simulink model "Test_driver"  (Simulink 7.6)
settings: Solver=ode45  StartTime=0.0  StopTime=10.0  RelTol=1e-3
undefined symbols (not defined in the file): Battery_Initial_Percentage, Battery_Nominal_Voltage, Battery_Size, Mass, Max_Engine_Power, Max_Engine_Torque
settings Model: Creator=Zsolt  LastModifiedBy=Zsolt
settings HardwareCC: TargetIntDivRoundTo=Zero  TargetEndianess=LittleEndian  TargetHWDeviceType=MATLAB Host  ProdEqTarget=off
settings RTWCC: SystemTargetFile=rsim.tlc  TemplateMakefile=rsim_default_tmf  Description=Rapid Simulation Target  ProcessScript=rsim_make_rtw_hook
settings RSimTargetCC: TargetFunctionLibrary=ANSI_C  ERTMultiwordTypeDef=System defined  ERTCodeCoverageTool=None  ERTMultiwordLength=256  IsPILTarget=off  EnableShiftOperators=on  PortableWordSizes=off

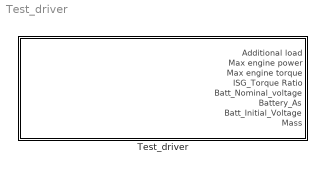
== system Test_driver ==
  Test_driver : Subsystem

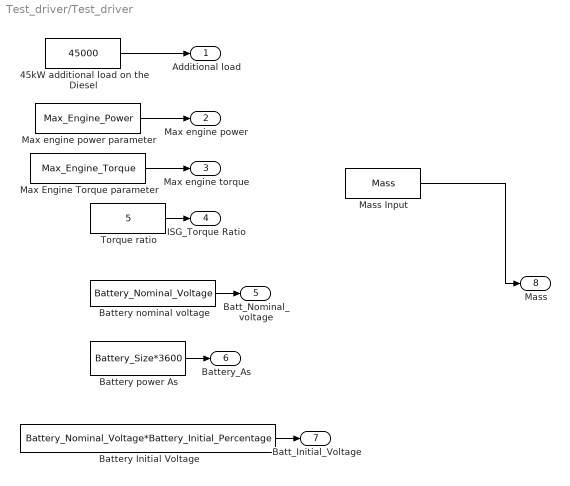
== system Test_driver/Test_driver ==
  45kW additional load on the Diesel : Constant  Value=45000
  Battery Initial Voltage : Constant  Value=Battery_Nominal_Voltage*Battery_Initial_Percentage
  Battery nominal voltage : Constant  Value=Battery_Nominal_Voltage
  Battery power As : Constant  Value=Battery_Size*3600
  Mass Input : Constant  Value=Mass
  Max Engine Torque parameter : Constant  Value=Max_Engine_Torque
  Max engine power parameter : Constant  Value=Max_Engine_Power
  Torque ratio : Constant  Value=5
  Additional load : Outport
  Max engine power : Outport  Port=2
  Max engine torque : Outport  Port=3
  ISG_Torque Ratio : Outport  Port=4
  Batt_Nominal_voltage : Outport  Port=5
  Battery_As : Outport  Port=6
  Batt_Initial_Voltage : Outport  Port=7
  Mass : Outport  Port=8
  wires:
  45kW additional load on the Diesel/1 -> Additional load/1
  Max engine power parameter/1 -> Max engine power/1
  Max Engine Torque parameter/1 -> Max engine torque/1
  Torque ratio/1 -> ISG_Torque Ratio/1
  Battery nominal voltage/1 -> Batt_Nominal_voltage/1
  Battery power As/1 -> Battery_As/1
  Battery Initial Voltage/1 -> Batt_Initial_Voltage/1
  Mass Input/1 -> Mass/1
